simulink subsystem "im_foc_decouple"  (R2022b)
settings: Solver=VariableStepAuto  StartTime=0.0  StopTime=10.0  RelTol=1e-3
settings Model: Creator=jack  LastModifiedBy=jack

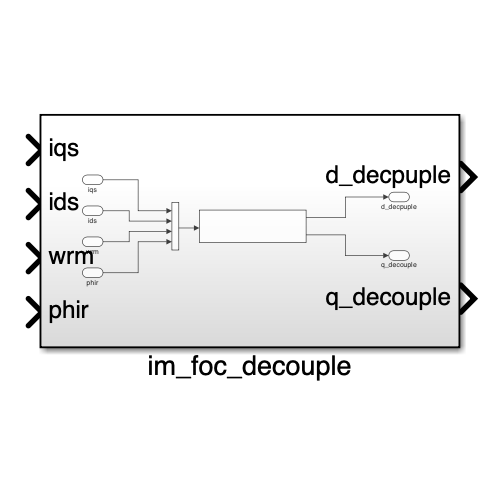
[thumbnail: Simulink's stored preview of the top-level diagram]
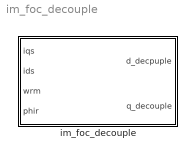
== system im_foc_decouple ==
  im_foc_decouple : Subsystem

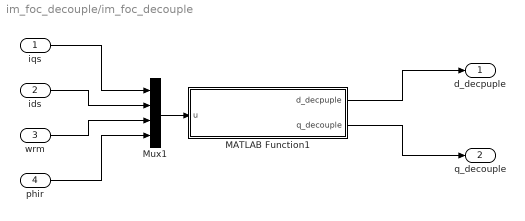
== system im_foc_decouple/im_foc_decouple ==
  iqs : Inport
  ids : Inport  Port=2
  wrm : Inport  Port=3
  phir : Inport  Port=4
  MATLAB Function1 : MATLAB Function  TreatAsAtomicUnit=on
  Mux1 : Mux
  d_decpuple : Outport
  q_decouple : Outport  Port=2
  wires:
  iqs/1 -> Mux1/1
  ids/1 -> Mux1/2
  wrm/1 -> Mux1/3
  Mux1/1 -> MATLAB Function1/1(u)
  MATLAB Function1/1(d_decpuple) -> d_decpuple/1
  MATLAB Function1/2(q_decouple) -> q_decouple/1
  phir/1 -> Mux1/4

== matlab function im_foc_decouple/MATLAB Function1 ==
  data: u input; d_decpuple output; q_decouple output
function [d_decpuple, q_decouple] = decouple(u)
    Rr = 0.6;
    Lr = 0.085;
    Ls = 0.085;
    Lm = 0.082;
    sigma = 1 - Lm^2/(Ls*Lr);
    Tr = Lr/Rr;
    pole = 4;
    wslip = (u(1)*Rr)/(u(2)*Lr+1e-8);
    we = wslip + u(3)*pole/2;
    d_decpuple = we*u(1) + (1-sigma)/(sigma*Lm*Tr)*u(4);
    q_decouple = we*u(2) + (1-sigma)/(sigma*Lm)*we*u(4);
